simulink model "q_2"  (R2020a)
settings: Solver=VariableStepAuto  StartTime=0.0  StopTime=10.0  RelTol=1e-3
model workspace (MAT data in the model file):
  K1 = 36000
  K2 = 204034.4
  M1 = 600
  M2 = 90
  b = 1000
settings Model: Creator=Admin  LastModifiedBy=Admin

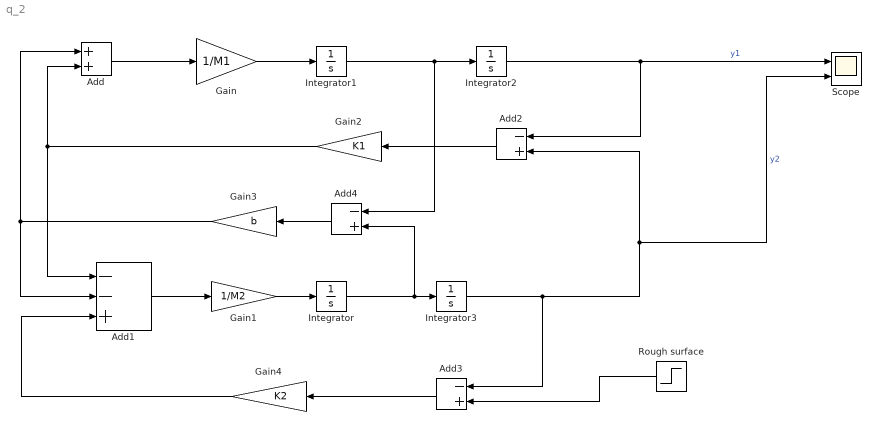
== system q_2 ==
  Add : Sum
  Add1 : Sum  Inputs=--+
  Add2 : Sum  Inputs=-+
  Add3 : Sum  Inputs=-+
  Add4 : Sum  Inputs=-+
  Gain : Gain  Gain=1/M1
  Gain1 : Gain  Gain=1/M2
  Gain2 : Gain  Gain=K1
  Gain3 : Gain  Gain=b
  Gain4 : Gain  Gain=K2
  Integrator{,1..3} (4 alike) : Integrator
  Rough surface : Step  SampleTime=0
  Scope : Scope  NumInputPorts=2
  wires:
  Integrator1/1 -> Integrator2/1, Add4/1
  Add/1 -> Gain/1
  Gain/1 -> Integrator1/1
  Integrator2/1 -> Scope/1, Add2/1  "y1"
  Gain1/1 -> Integrator/1
  Add1/1 -> Gain1/1
  Integrator/1 -> Add4/2, Integrator3/1
  Integrator3/1 -> Add3/1, Scope/2, Add2/2  "y2"
  Add2/1 -> Gain2/1
  Gain2/1 -> Add1/1, Add/2
  Gain3/1 -> Add/1, Add1/2
  Rough surface/1 -> Add3/2
  Gain4/1 -> Add1/3
  Add4/1 -> Gain3/1
  Add3/1 -> Gain4/1
